simulink model "F16_Sim"  (R2025a)
settings: Solver=VariableStepAuto  StartTime=0.0  StopTime=10.0  RelTol=1e-3
values from neighbouring files (symbols this model uses):
  U = [10; 2; 0; 5; 2; 20]    [main.m]
  Y0 = [100; 4; 1; 0.1; 0.05; 0.08; 5; 0; 10; 0; 0; -200]    [main.m]
settings Model: Creator=deepa  LastModifiedBy=deepa

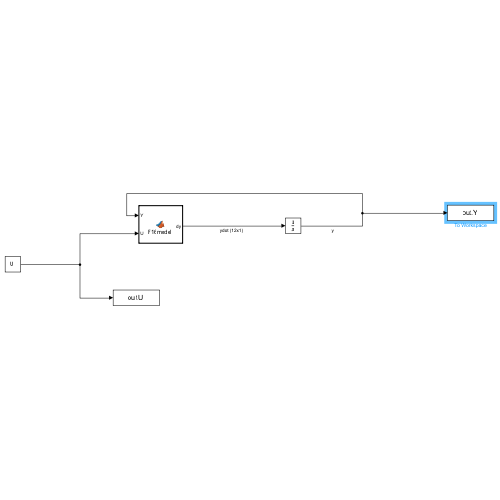
[thumbnail: Simulink's stored preview of the top-level diagram]
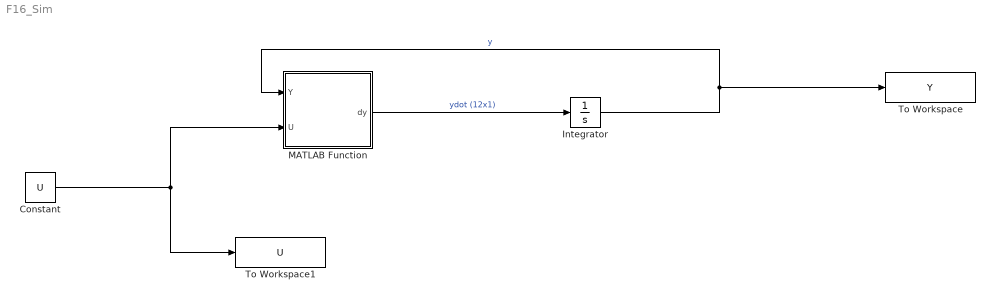
== system F16_Sim ==
  Constant : Constant  Value=U
  Integrator : Integrator  InitialCondition=Y0
  MATLAB Function : MATLAB Function  TreatAsAtomicUnit=on
  To Workspace : ToWorkspace  VariableName=Y  SaveFormat=Timeseries  SampleTime=-1
  To Workspace1 : ToWorkspace  VariableName=U  SaveFormat=Timeseries  SampleTime=-1
  wires:
  MATLAB Function/1(dy) -> Integrator/1  "ydot (12x1)"
  Integrator/1 -> MATLAB Function/1(Y), To Workspace/1  "y"
  Constant/1 -> To Workspace1/1, MATLAB Function/2(U)

== matlab function F16_Sim/MATLAB Function ==
  data: Y input; dy output; U input
function dy = F16model(Y,U)


    % State variables
    u = Y(1); % y1
    v = Y(2); % y2
    w = Y(3); % y3
    
    p = Y(4); % y4
    q = Y(5); % y5
    r = Y(6); % y6

    phi = deg2rad(Y(7));   % Roll angle (rad)
    theta = deg2rad(Y(8)); % Pitch angle (rad)
    psi = deg2rad(Y(9)); % Yaw angle (rad)

    xpos = Y(10);  % X position (m)
    ypos = Y(11);  % Y position (m)
    zpos = Y(12);  % Z position (m, positive downward)

    del_A = U(1);
    del_R = U(2);
    del_E = U(3);
    del_LEF = U(4);
    del_SB = U(5);
    thrtl = U(6);

    V_t = sqrt(u^2 + v^2 + w^2);
    alpha = atan2(w,u); % Angle of attack (rad)
    beta = asin(v/V_t);  % Sideslip angle (rad)
    

    m = 8936;
    Ixx = 12896;
    Iyy = 75800;
    Izz = 85672;
    Ixz = 1332;
    b = 9.96;
    S = 27.87;
    c = 3.45;
    x_cg_ref = 0.35*c;
    x_cg = 0.38*c;

    g = 9.81;
    H_e = 216.9; % Engine Angular Momentum kg-m^2/sec
    % Compute air data
    rho = 1.225;
    qbar = 0.5*rho*(V_t)^2;     % Dynamic pressure

   
    
    
    % Compute aerodynamic coefficients
    
    Cx =  -0.032 - 0.08*alpha - 0.02*del_E; % Longitudinal force coefficient
    Cy = -0.57*beta + 0.05*(del_R/30); % Normal force coefficient
    Cz = -0.34 - 1.8*alpha - 0.2*del_E;
    Cl = -0.02*beta + 0.15*(del_A/20) + 0.02*(del_R/30); % Roll moment coefficient
    Cm = 0.05 - 0.21*alpha - 0.5*del_E; % Pitch moment coefficient
    Cn = 0.057*beta + 0.01*(del_A/20) + 0.19*(del_R/30); % Yaw moment coefficient
    
    % Velocity components in body frame
    
    % Thrust (simplified as zero for this model)
    T = thrtl*m*g;         % Thrust force (N)
    %sigmaT = 0;    % Thrust angle (rad)
    
    % Force equations (acceleration in body frame)
    udot = -(q * w) + (r * v) - (g * sin(theta)) + (qbar * S * Cx) / m + (T/m);
    vdot = -(r * u) + (p * w) + (g * cos(theta) * sin(phi)) + ((qbar*S)/m)*Cy;
    wdot = -(p * v) + (q * u) + (g * cos(theta) * cos(phi)) + (qbar * S * Cz) / m;
    
    % Moment equations (angular acceleration)
    pdot = (qbar * S * b * (Izz * Cl + Ixz * Cn) - q * r * (Ixz^2 + Izz^2 + Iyy * Izz) + p * q * Ixz * (Ixx - Iyy + Izz)) / ((Ixx * Izz) - (Ixz^2)) - (H_e * r);
    qdot = (qbar * S * c * Cm - (p^2 - r^2) * Ixz + p * r * (Izz - Ixx)) / Iyy;
    rdot = ((qbar * S * b * (Ixx * Cn + Ixz * Cl) - q * r * (Ixx - Iyy + Izz) + p * q * (Ixz^2 + Ixx^2 - Ixx * Iyy)) / (Ixx * Izz - Ixz^2)) + (H_e * q);
    
    % Euler angle rates
    phidot = p + q * tan(theta) * sin(phi) + r * tan(theta) * cos(phi);
    thetadot = q * cos(phi) - r * sin(phi);
    psidot = (r * cos(phi) + q * sin(phi)) * sec(theta);
    
    % Position rates in inertial frame
    xdot = u * cos(theta) * cos(psi) + v * (sin(phi) * sin(theta) * cos(psi) - cos(phi) * sin(psi)) + w * (cos(phi) * sin(theta) * cos(psi) + sin(phi) * sin(psi));
    ydot = u * cos(theta) * sin(psi) + v * (sin(phi) * sin(theta) * sin(psi) + cos(phi) * cos(psi)) + w * (cos(phi) * sin(theta) * sin(psi) - sin(phi) * cos(psi));
    zdot = -u * sin(theta) + v * sin(phi) * cos(theta) + w * cos(phi) * cos(theta);
    
    % State derivative vector
    dy = [udot; vdot; wdot; pdot; qdot; rdot; phidot; thetadot; psidot; xdot; ydot; zdot];
end
